simulink model "practica5simulink"  (R2014a)
settings: Solver=ode45  StartTime=0.0  StopTime=0.1  RelTol=1e-3
values from neighbouring files (symbols this model uses):
  C = 1*10^-6    (= 1e-06)    [practica5matlab.m]
  R = 4.7*10^3    (= 4700)    [practica5matlab.m]
  v = 5    [practica5matlab.m]
settings Model: Creator=Diana  LastModifiedBy=Diana

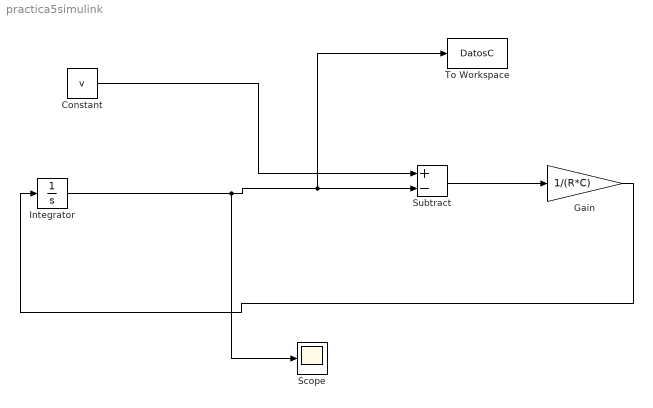
== system practica5simulink ==
  Constant : Constant  Value=v
  Gain : Gain  Gain=1/(R*C)
  Integrator : Integrator
  Scope : Scope
      settings: TimeRange=0.02
  Subtract : Sum  Inputs=+-
  To Workspace : ToWorkspace  VariableName=DatosC  SaveFormat=Timeseries  SampleTime=-1
  wires:
  Constant/1 -> Subtract/1
  Subtract/1 -> Gain/1
  Gain/1 -> Integrator/1
  Integrator/1 -> Scope/1, To Workspace/1, Subtract/2
